simulink model "VehicleDynamicsRing"  (R2020a)
settings: Solver=FixedStepDiscrete  StartTime=0.0  StopTime=10.0  FixedStep=ModelSimTime  RelTol=1e-3  EnableMultiTasking=on
PostLoadFcn:
  | , if any(exist('dsrtsu_mdlpostloadfcn', 'file') ~= 0), dsrtsu_mdlpostloadfcn('Execute', bdroot); end,
InitFcn:
  | , if any(exist('rtifpga_mdlclblib', 'file') ~= 0), rtifpga_mdlclblib('Init', bdroot); end,
undefined symbols (not defined in the file): DRIVE_MODE, VDR
libraries: simulink x4
(part 2 of 2)

== stateflow chart VehicleDynamicsRing/VDR Mode Selection1 ==
  state VDR_MASTER
    state MODES [parallel]
      settings: executionOrder=1
      state OFF
        during:
        TVEnable = 0;
        UnstblEnable = 0;
        OpenDiffEnable = 0;
        AWDEnable = 0;
        FWDEnable = 0;
        RWDEnable = 0 ;
        MotorStatus = [0,0,0,0];
        DriveEnable = 0;
        StartUpTest = 0;
        Status = VDR.OFF;
        APPS_Status = VDR.ERROR.APPS.OKAY;
      state STARTUP
        entry:
        StartUpTestCheck();
        TVEnable = 1;
        UnstblEnable = 1;
        OpenDiffEnable = 1;
        AWDEnable = 1;
        FWDEnable = 1;
        RWDEnable = 1;
        MotorStatus = [1,1,1,1];
        Status = VDR.STARTUP;
      state SHUTDOWN
        entry:
        DriveEnable = 0;
        Status = VDR.SHUTDOWN;
      state DRIVING
        entry:
        DriveEnable = 1;
        Status = VDR.DRIVING;
      (default) -> OFF
      OFF -> STARTUP : E_StartUp
      SHUTDOWN -> OFF : E_Off
      STARTUP -> SHUTDOWN [order 2] : E_FailStartUp
      DRIVING -> SHUTDOWN : E_ShutDown
      STARTUP -> DRIVING [order 1] : E_Driving
    state CHECKING_SENSORS_ERRORS_AND_DIAGNOSTICS [parallel]
      settings: executionOrder=2
      state WAITING_TO_CHECK_SENSORS
        entry:
      state CHECKING_SENSORS
        during:
        CheckingSensorsTable();
      (default) -> WAITING_TO_CHECK_SENSORS
      WAITING_TO_CHECK_SENSORS -> CHECKING_SENSORS : E_Driving
    state MODE_SELECTION_LOGIC [parallel]
      settings: executionOrder=3
      state STANDBY
        entry:
      state CHECK_MODE_CHANGE
        %Check for valid mode
      state VALID_MODE
      state CHANGE_MAIN_MODE
        entry:
        ChangeMainMode();
      state DENY_DRIVING_MODE
        entry:
        %Cannot start driving the vehicle yet
        %First need to startup the car and run tests.
        %Send out status
      state VALID_DRIVING_MODE
      state DENY_DRIVING_MODE_CHANGE1
        %Envalid mode status
      state CHECK_DRIVING_MODE_CHANGE
      state DENY_DRIVING_MODE_CHANGE
        entry: %Deny and send out status
      state APPROVED_DRIVING_MODE_CHANGE
        entry: ChangeDrivingMode();
      state DriveModeCheck = ModeChecking [function]
        (junction 1413) -> (junction 1412)
        (junction 1412) -> (junction 1414)
        (junction 1417) -> (junction 1413) [order 3] : {ModeCheck = 0;}
            | %Else Deny
        (junction 1415) -> (junction 1414) [order 2]
        (junction 1416) -> (junction 1415) [order 1] : [sum(VDRMode == 10:12) == 1]
            | %Unstable Torque Vectoring
        (junction 1417) -> (junction 1416) [order 2] : [TVEnable == 1 && sum(VDRMode == 10:15) == 1]
            | %Torque Vecoting Check
        (default) -> (junction 1417) : %START
        (junction 1416) -> (junction 1418) [order 2] : %Else Stable Torque Vectoring
        (junction 1414) -> (junction 1426)
        (junction 1415) -> (junction 1418) [order 1] : [UnstblEnable == 1]
        (junction 1417) -> (junction 1419) [order 1] : [OpenDiffEnable == 1 && sum(VDRMode == 16:18) == 1]
            | %Open Differential Check
        (junction 1419) -> (junction 1418)
        (junction 1418) -> (junction 1420) : % Main Mode  request check passed
            | % Checking for drivetrain request
        (junction 1420) -> (junction 1421) [order 1] : [VDRMode == 10 || VDRMode == 13 || VDRMode == 16 && AWDEnable == 1]
            | %Checking for AWD
        (junction 1420) -> (junction 1422) [order 2]
        (junction 1421) -> (junction 1430) : {ModeCheck = 1;}
        (junction 1422) -> (junction 1423) [order 1] : [VDRMode == 11 || VDRMode == 14 || VDRMode == 17 && FWDEnable == 1]
            | %Checking for FWD
        (junction 1422) -> (junction 1424) [order 2]
        (junction 1423) -> (junction 1429) : {ModeCheck=1;}
        (junction 1424) -> (junction 1425) [order 1] : [VDRMode == 12 || VDRMode == 15 || VDRMode == 18 && RWDEnable == 1]
            | %Checking for FWD
        (junction 1424) -> (junction 1427) [order 2] : {ModeCheck=0;}
            | %Deny
        (junction 1425) -> (junction 1428) : {ModeCheck=1;}
        (junction 1426) -> (junction 1427) : {ModeCheck = 0}
            | %Else Deny
        (junction 1428) -> (junction 1427)
        (junction 1429) -> (junction 1428)
        (junction 1430) -> (junction 1429)
        (junction 1427) -> (junction 1431) : {DriveModeCheck = ModeCheck;}
            | %END
      state CheckStatus = ValidModeChecking [function]
        (default) -> (junction 1388) : %START
            | %Checking for a valid main mode
        (junction 1388) -> (junction 1389) [order 1] : [sum(VDRMode == 0:3) == 1]
            | %Check for main modes
        (junction 1388) -> (junction 1390) [order 2]
        (junction 1389) -> (junction 1395) : {ValidModeCheck=1;}
        (junction 1390) -> (junction 1391) [order 1] : [sum(VDRMode == 10:18) == 1]
            | %Check for driving modes
        (junction 1390) -> (junction 1392) [order 2] : {ValidModeCheck=0;}
            | %Else: Invalid Mode
        (junction 1391) -> (junction 1394) : {ValidModeCheck=1;}
        (junction 1393) -> (junction 1392)
        (junction 1394) -> (junction 1393)
        (junction 1395) -> (junction 1394)
        (junction 1392) -> (junction 1396) : {CheckStatus =ValidModeCheck; }
            | %END
      (junction 982) -> (junction 983)
      (junction 983) -> STANDBY
      (junction 981) -> (junction 982)
      (default) -> STANDBY
      CHECK_MODE_CHANGE -> VALID_MODE [order 1] : [ValidModeChecking()]
      VALID_MODE -> CHANGE_MAIN_MODE [order 2]
      CHANGE_MAIN_MODE -> (junction 981)
      STANDBY -> CHECK_MODE_CHANGE : [hasChanged(VDRMode)]
      (junction 980) -> (junction 981)
      CHECK_MODE_CHANGE -> DENY_DRIVING_MODE_CHANGE1 [order 2]
      VALID_MODE -> VALID_DRIVING_MODE [order 1] : [sum(VDRMode == 10:18) ==1]
      VALID_DRIVING_MODE -> DENY_DRIVING_MODE [order 2]
      DENY_DRIVING_MODE -> (junction 980)
      (junction 979) -> (junction 980)
      VALID_DRIVING_MODE -> CHECK_DRIVING_MODE_CHANGE [order 1] : [StartUpTest == 1]
      CHECK_DRIVING_MODE_CHANGE -> DENY_DRIVING_MODE_CHANGE [order 2]
      DENY_DRIVING_MODE_CHANGE -> (junction 979)
      (junction 984) -> (junction 979)
      CHECK_DRIVING_MODE_CHANGE -> APPROVED_DRIVING_MODE_CHANGE [order 1] : [ModeChecking()]
      APPROVED_DRIVING_MODE_CHANGE -> (junction 984)
    state MOTOR_STATUSES [parallel]
      entry:
      encoder_torque_counter_FL = 0;
      encoder_torque_counter_FR = 0;
      encoder_torque_counter_RL = 0;
      encoder_torque_counter_RR = 0;
      acceleration_torque_counter_FL = 0;
      acceleration_torque_counter_FR = 0;
      acceleration_torque_counter_RL = 0;
      acceleration_torque_counter_RR = 0;
      settings: executionOrder=4
      state MOTOR_STATUS_FL [parallel] [commented out]
        state MOTOR_CHECKING_FL [commented out]
          state MOTOR_ENCODER_CHECK_FL [parallel] [commented out]
            state CHECKING_ENC_FL [commented out]
              during:
              encoder_torque_counter_FL = duration_encoder_torque_check(SystemTrqCmd ,Encoder_FL,encoder_torque_counter_FL);
            state ENC_ERR_FL [commented out]
              en:
              send(E_MtrErrFL,MOTOR_STATUS_FL)
            (default) -> CHECKING_ENC_FL [commented out]
            CHECKING_ENC_FL -> ENC_ERR_FL [commented out] : [encoder_torque_counter_FL >= VDR.EncoderTorqueCounter]
          state MOTOR_ACCEL_CHECK_FL [parallel] [commented out]
            state ERR_ACCEL_FL [commented out]
              en:
              send(E_MtrErrFL,MOTOR_STATUS_FL)
            state CHECKING_ACCEL_FL [commented out]
              during:
              acceleration_torque_counter_FL = duration_acceleration_torque_check(SystemTrqCmd ,Accel_X,acceleration_torque_counter_FL);
            (default) -> CHECKING_ACCEL_FL [commented out]
            CHECKING_ACCEL_FL -> ERR_ACCEL_FL [commented out] : [acceleration_torque_counter_FL >= VDR.AccelTorqueCounter]
          state MOTOR_TRQ_LIMIT_CHECK_FL [parallel] [commented out]
            state CHECKING_TRQ_LIMIT_FL [commented out]
            state ERR_TRQ_LIMIT_FL [commented out]
              en:
              send(E_MtrErrFL,MOTOR_STATUS_FL)
            (default) -> CHECKING_TRQ_LIMIT_FL [commented out]
            CHECKING_TRQ_LIMIT_FL -> ERR_TRQ_LIMIT_FL [commented out] : [TorqueLimit_FL > 21 || TorqueLimit_FL < 0]
          state MOTOR_ENCODER_VALUE_CHECK_FL [parallel] [commented out]
            state CHECKING_ENCODER_VALUE_FL [commented out]
            state ERR_ENCODER_VALUEL_FL [commented out]
              en:
              send(E_MtrErrFL,MOTOR_STATUS_FL)
            (default) -> CHECKING_ENCODER_VALUE_FL [commented out]
            CHECKING_ENCODER_VALUE_FL -> ERR_ENCODER_VALUEL_FL [commented out] : [Encoder_FL > 7000]
        state FWD_OFF_FL [commented out]
          entry:
          %nothing
        state MTR_ERR_FL [commented out]
          entry:
          %send status
          FWDEnable = 0;
        (default) -> MOTOR_CHECKING_FL [commented out]
        MOTOR_CHECKING_FL -> FWD_OFF_FL [commented out] : [FWDEnable == 0]
        MOTOR_CHECKING_FL -> MTR_ERR_FL [commented out] : E_MtrErrFL
      state MOTOR_STATUS_FR [parallel] [commented out]
        state MOTOR_CHECKING_FR [commented out]
          state MOTOR_ENCODER_CHECK_FR [parallel] [commented out]
            state CHECKING_ENC_FR [commented out]
              during:
              encoder_torque_counter_FR = duration_encoder_torque_check(SystemTrqCmd ,Encoder_FR,encoder_torque_counter_FR);
            state ENC_ERR_FR [commented out]
              en:
              send(E_MtrErrFR,MOTOR_STATUS_FR)
            (default) -> CHECKING_ENC_FR [commented out]
            CHECKING_ENC_FR -> ENC_ERR_FR [commented out] : [encoder_torque_counter_FR >= VDR.EncoderTorqueCounter]
          state MOTOR_ACCEL_CHECK_FR [parallel] [commented out]
            state ERR_ACCEL_FR [commented out]
              en:
              send(E_MtrErrFR,MOTOR_STATUS_FR)
            state CHECKING_ACCEL_FR [commented out]
              during:
              acceleration_torque_counter_FR = duration_acceleration_torque_check(SystemTrqCmd ,Accel_X,acceleration_torque_counter_FR);
            (default) -> CHECKING_ACCEL_FR [commented out]
            CHECKING_ACCEL_FR -> ERR_ACCEL_FR [commented out] : [acceleration_torque_counter_FR >= VDR.AccelTorqueCounter]
          state MOTOR_TRQ_LIMIT_CHECK_FR [parallel] [commented out]
            state CHECKING_TRQ_LIMIT_FR [commented out]
            state ERR_TRQ_LIMIT_FR [commented out]
              en:
              send(E_MtrErrFR,MOTOR_STATUS_FR)
            (default) -> CHECKING_TRQ_LIMIT_FR [commented out]
            CHECKING_TRQ_LIMIT_FR -> ERR_TRQ_LIMIT_FR [commented out] : [TorqueLimit_FR > 21 || TorqueLimit_FR < 0]
          state MOTOR_ENCODER_VALUE_CHECK_FR [parallel] [commented out]
            state CHECKING_ENCODER_VALUE_FR [commented out]
            state ERR_ENCODER_VALUEL_FR [commented out]
              en:
              send(E_MtrErrFR,MOTOR_STATUS_FR)
            (default) -> CHECKING_ENCODER_VALUE_FR [commented out]
            CHECKING_ENCODER_VALUE_FR -> ERR_ENCODER_VALUEL_FR [commented out] : [Encoder_FR > 7000]
        state FWD_OFF_FR [commented out]
          entry:
          %nothing
        state MTR_ERR_FR [commented out]
          entry:
          %send status
          FWDEnable = 0;
        (default) -> MOTOR_CHECKING_FR [commented out]
        MOTOR_CHECKING_FR -> FWD_OFF_FR [commented out] : [FWDEnable == 0]
        MOTOR_CHECKING_FR -> MTR_ERR_FR [commented out] : E_MtrErrFR
      state MOTOR_STATUS_RL [parallel] [commented out]
        state MOTOR_CHECKING_RL [commented out]
          state MOTOR_ENCODER_CHECK_RL [parallel] [commented out]
            state CHECKING_ENC_RL [commented out]
              during:
              encoder_torque_counter_RL = duration_encoder_torque_check(SystemTrqCmd ,Encoder_RL,encoder_torque_counter_RL);
            state ENC_ERR_RL [commented out]
              en:
              send(E_MtrErrRL,MOTOR_STATUS_RL)
            (default) -> CHECKING_ENC_RL [commented out]
            CHECKING_ENC_RL -> ENC_ERR_RL [commented out] : [encoder_torque_counter_RL >= VDR.EncoderTorqueCounter]
          state MOTOR_ACCEL_CHECK_RL [parallel] [commented out]
            state ERR_ACCEL_RL [commented out]
              en:
              send(E_MtrErrRL,MOTOR_STATUS_RL)
            state CHECKING_ACCEL_RL [commented out]
              during:
              acceleration_torque_counter_RL = duration_acceleration_torque_check(SystemTrqCmd ,Accel_X,acceleration_torque_counter_RL);
            (default) -> CHECKING_ACCEL_RL [commented out]
            CHECKING_ACCEL_RL -> ERR_ACCEL_RL [commented out] : [acceleration_torque_counter_RL >= VDR.AccelTorqueCounter]
          state MOTOR_TRQ_LIMIT_CHECK_RL [parallel] [commented out]
            state CHECKING_TRQ_LIMIT_RL [commented out]
            state ERR_TRQ_LIMIT_RL [commented out]
              en:
              send(E_MtrErrRL,MOTOR_STATUS_RL)
            (default) -> CHECKING_TRQ_LIMIT_RL [commented out]
            CHECKING_TRQ_LIMIT_RL -> ERR_TRQ_LIMIT_RL [commented out] : [TorqueLimit_RL > 21 || TorqueLimit_RL < 0]
          state MOTOR_ENCODER_VALUE_CHECK_RL [parallel] [commented out]
            state CHECKING_ENCODER_VALUE_RL [commented out]
            state ERR_ENCODER_VALUEL_RL [commented out]
              en:
              send(E_MtrErrRL,MOTOR_STATUS_RL)
            (default) -> CHECKING_ENCODER_VALUE_RL [commented out]
            CHECKING_ENCODER_VALUE_RL -> ERR_ENCODER_VALUEL_RL [commented out] : [Encoder_RL > 7000]
        state FWD_OFF_RL [commented out]
          entry:
          %nothing
        state MTR_ERR_RL [commented out]
          entry:
          %send status
          FWDEnable = 0;
        (default) -> MOTOR_CHECKING_RL [commented out]
        MOTOR_CHECKING_RL -> FWD_OFF_RL [commented out] : [FWDEnable == 0]
        MOTOR_CHECKING_RL -> MTR_ERR_RL [commented out] : E_MtrErrRL
      state MOTOR_STATUS_RR [parallel] [commented out]
        state MOTOR_CHECKING_RR [commented out]
          state MOTOR_ENCODER_CHECK_RR [parallel] [commented out]
            state CHECKING_ENC_RR [commented out]
              during:
              encoder_torque_counter_RR = duration_encoder_torque_check(SystemTrqCmd ,Encoder_RR,encoder_torque_counter_RR);
            state ENC_ERR_RR [commented out]
              en:
              send(E_MtrErrRR,MOTOR_STATUS_RR)
            (default) -> CHECKING_ENC_RR [commented out]
            CHECKING_ENC_RR -> ENC_ERR_RR [commented out] : [encoder_torque_counter_RR >= VDR.EncoderTorqueCounter]
          state MOTOR_ACCEL_CHECK_RR [parallel] [commented out]
            state ERR_ACCEL_RR [commented out]
              en:
              send(E_MtrErrRR,MOTOR_STATUS_RR)
            state CHECKING_ACCEL_RR [commented out]
              during:
              acceleration_torque_counter_RR = duration_acceleration_torque_check(SystemTrqCmd ,Accel_X,acceleration_torque_counter_RR);
            (default) -> CHECKING_ACCEL_RR [commented out]
            CHECKING_ACCEL_RR -> ERR_ACCEL_RR [commented out] : [acceleration_torque_counter_RR >= VDR.AccelTorqueCounter]
          state MOTOR_TRQ_LIMIT_CHECK_RR [parallel] [commented out]
            state CHECKING_TRQ_LIMIT_RR [commented out]
            state ERR_TRQ_LIMIT_RR [commented out]
              en:
              send(E_MtrErrRR,MOTOR_STATUS_RR)
            (default) -> CHECKING_TRQ_LIMIT_RR [commented out]
            CHECKING_TRQ_LIMIT_RR -> ERR_TRQ_LIMIT_RR [commented out] : [TorqueLimit_RR > 21 || TorqueLimit_RR < 0]
          state MOTOR_ENCODER_VALUE_CHECK_RR [parallel] [commented out]
            state CHECKING_ENCODER_VALUE_RR [commented out]
            state ERR_ENCODER_VALUEL_RR [commented out]
              en:
              send(E_MtrErrRR,MOTOR_STATUS_RR)
            (default) -> CHECKING_ENCODER_VALUE_RR [commented out]
            CHECKING_ENCODER_VALUE_RR -> ERR_ENCODER_VALUEL_RR [commented out] : [Encoder_RR > 7000]
        state FWD_OFF_RR [commented out]
          entry:
          %nothing
        state MTR_ERR_RR [commented out]
          entry:
          %send status
          FWDEnable = 0;
        (default) -> MOTOR_CHECKING_RR [commented out]
        MOTOR_CHECKING_RR -> FWD_OFF_RR [commented out] : [FWDEnable == 0]
        MOTOR_CHECKING_RR -> MTR_ERR_RR [commented out] : E_MtrErrRR
      state updated_counter = duration_encoder_torque_check(trq,encoder,counter) [function]
      state updated_counter = duration_acceleration_torque_check(trq,accel,counter) [function]
  (default) -> VDR_MASTER
  data: DriveModeCheck function_output; CheckStatus function_output; trq function_input double size=1; encoder function_input double size=1; counter function_input double size=1; updated_counter function_output; trq function_input double size=1; accel function_input double size=1; counter function_input double size=1; updated_counter function_output; VDRMode input; VDR parameter; TVEnable local; UnstblEnable local; OpenDiffEnable local; AWDEnable local; FWDEnable local; RWDEnable local; MotorStatus local; APPS1 input; APPS2 input; Accel_X input; Accel_Y input; Speed_X input; Speed input; SteerAngle input; APPS input; Encoder_FL input; Encoder_FR input; Encoder_RL input; Encoder_RR input; SystemTrqCmd input; TorqueLimit_FL input; TorqueLimit_FR input; TorqueLimit_RL input; TorqueLimit_RR input; ValidModeCheck local; encoder_torque_counter_FL local double; acceleration_torque_counter_FL local double; acceleration_torque_counter_RL local double; acceleration_torque_counter_RR local double; encoder_torque_counter_RR local double; encoder_torque_counter_FR local double; encoder_torque_counter_RL local double; acceleration_torque_counter_FR local double; DrivingMode output; TVControl output; Drivetrain output; DriveEnable output; Status output; APPS_Status output; StartUpTest local
  events: E_StartUp local FUNCTION_CALL_EVENT; E_ShutDown local FUNCTION_CALL_EVENT; E_Off local FUNCTION_CALL_EVENT; E_FailStartUp local FUNCTION_CALL_EVENT; E_Driving local FUNCTION_CALL_EVENT; E_MtrErrRR local FUNCTION_CALL_EVENT; E_MtrErrFL local FUNCTION_CALL_EVENT; E_MtrErrFR local FUNCTION_CALL_EVENT; E_MtrErrRL local FUNCTION_CALL_EVENT; E_CommunicationCheck local RISING_EDGE_EVENT
  function StartUpTestCheck:
    | function StartUpTestCheck
    | 
    | aVarTruthTableCondition_1 = false;
    | aVarTruthTableCondition_2 = false;
    | aVarTruthTableCondition_3 = false;
    | aVarTruthTableCondition_4 = false;
    | aVarTruthTableCondition_5 = false;
    | aVarTruthTableCondition_6 = false;
    | 
    | 
    | % Look at APPS
    | 
    | aVarTruthTableCondition_1 = logical(APPS >= 0 && APPS <= 100);
    | 
    | % Car is not moving check: accel-x
    | 
    | aVarTruthTableCondition_2 = logical(abs(Accel_X) < VDR.MinAccelX);
    | 
    | % Car is not moving check: accel-y
    | 
    | aVarTruthTableCondition_3 = logical(abs(Accel_Y) < VDR.MinAccelY);
    | 
    | % Velocity-x sensor is zero
    | 
    | aVarTruthTableCondition_4 = logical(abs(Speed_X) < VDR.MinVelocityX);
    | 
    | % Velocity sensor is zero
    | 
    | aVarTruthTableCondition_5 = logical(abs(Speed) < VDR.MinVelocity);
    | 
    | % Check Steering Wheel calibr.
    | 
    | aVarTruthTableCondition_6 = logical(abs(SteerAngle) < VDR.MaxSteerAngle);
    | 
    | if (aVarTruthTableCondition_1 && aVarTruthTableCondition_2 && aVarTruthTableCondition_3 && aVarTruthTableCondition_4 && aVarTruthTableCondition_5 && aVarTruthTableCondition_6)
    |     aFcnTruthTableAction_1();
    | else % Default
    |     aFcnTruthTableAction_2();
    | end
    | 
    | function aFcnTruthTableAction_1()
    | 
    | % The car is stationary and can now be started up.
    | 
    | StartUpTest = 1;
    | 
    | function aFcnTruthTableAction_2()
    | 
    | % The car sensors readons are incorrect or the car is moving. So the car should not be started up.
    | 
    | send(E_FailStartUp,MODES);
  function CheckingSensorsTable:
    | function CheckingSensorsTable
    | 
    | aVarTruthTableCondition_1 = false;
    | aVarTruthTableCondition_2 = false;
    | aVarTruthTableCondition_3 = false;
    | aVarTruthTableCondition_4 = false;
    | aVarTruthTableCondition_5 = false;
    | 
    | 
    | % Steering sensor sanity check
    | 
    | aVarTruthTableCondition_1 = logical(abs(SteerAngle) > VDR.MaxSteerAngle);
    | 
    | % System Command Torque Check
    | 
    | aVarTruthTableCondition_2 = logical(abs(SystemTrqCmd) > 90);
    | 
    | % APPS competition requirements
    | 
    | aVarTruthTableCondition_3 = logical(abs(APPS1 - APPS2)/APPS1 >= 0.1);
    | 
    | % Accelerator-x sanity check
    | 
    | aVarTruthTableCondition_4 = logical(abs(Accel_X) > VDR.MaxAccelX);
    | 
    | % Accelerator-y sanity check
    | 
    | aVarTruthTableCondition_5 = logical(abs(Accel_Y) > VDR.MaxAccelY);
    | 
    | if (aVarTruthTableCondition_1)
    |     aFcnTruthTableAction_1();
    |     aFcnTruthTableAction_3();
    | elseif (aVarTruthTableCondition_2)
    |     aFcnTruthTableAction_1();
    | elseif (aVarTruthTableCondition_3)
    |     aFcnTruthTableAction_1();
    |     aFcnTruthTableAction_2();
    | elseif (aVarTruthTableCondition_4)
    |     aFcnTruthTableAction_3();
    | elseif (aVarTruthTableCondition_5)
    |     aFcnTruthTableAction_3();
    | else % Default
    |     aFcnTruthTableAction_1();
    | end
    | 
    | function aFcnTruthTableAction_1()
    | 
    | % Impossible and/or out of range values. Must shutdown the vehicle.
    | 
    | send(E_ShutDown,MODES);
    | 
    | function aFcnTruthTableAction_2()
    | 
    | % APPS Failure
    | 
    | APPS_Status = VDR.ERROR.APPS.FAILURE;
    | 
    | function aFcnTruthTableAction_3()
    | 
    | % Disable the unstable Torque Vectoring controller
    | 
    | UnstblEnable = 0;
  function ChangeMainMode:
    | function ChangeMainMode
    | switch(VDRMode)
    |     case VDR.Mode.OFF
    |         send(E_Off,MODES);
    |     case VDR.Mode.STARTUP
    |         send(E_StartUp,MODES);
    |     case VDR.Mode.DRIVING
    |         send(E_Driving,MODES);
    |     case VDR.Mode.SHUTDOWN
    |         send(E_ShutDown,MODES);
    |     otherwise
    |         send(E_ShutDown,MODES);
    | end
  function ChangeMainMode12:
    | function ChangeMainMode12
    | 
    | aVarTruthTableCondition_1 = false;
    | aVarTruthTableCondition_2 = false;
    | aVarTruthTableCondition_3 = false;
    | aVarTruthTableCondition_4 = false;
    | 
    | 
    | % Startup requested
    | 
    | aVarTruthTableCondition_1 = logical(VDRMode == 0);
    | 
    | % Shutdown requested
    | 
    | aVarTruthTableCondition_2 = logical(VDRMode == 1);
    | 
    | % Driving requested
    | 
    | aVarTruthTableCondition_3 = logical(VDRMode == 2);
    | 
    | % OFF requested
    | 
    | aVarTruthTableCondition_4 = logical(VDRMode == 3);
    | 
    | if (aVarTruthTableCondition_1)
    |     aFcnTruthTableAction_1();
    | elseif (aVarTruthTableCondition_2)
    |     aFcnTruthTableAction_2();
    | elseif (aVarTruthTableCondition_3)
    |     aFcnTruthTableAction_3();
    | elseif (aVarTruthTableCondition_4)
    |     aFcnTruthTableAction_4();
    | else % Default
    |     aFcnTruthTableAction_4();
    | end
    | 
    | function aFcnTruthTableAction_1()
    | 
    | % Switch to Startup
    | 
    | send(E_StartUp,MODES);
    | 
    | function aFcnTruthTableAction_2()
    | 
    | % Switch to Shutdown
    | 
    | send(E_Off,MODES);
    | 
    | function aFcnTruthTableAction_3()
    | 
    | % Switch to OFF
    | 
    | send(E_Driving,MODES);
    | 
    | function aFcnTruthTableAction_4()
    | 
    | % Error in mode selection.
    | 
    | send(E_ShutDown,MODES);
  function ChangeDrivingMode:
    | function ChangeDrivingMode
    | 
    | aVarTruthTableCondition_1 = false;
    | aVarTruthTableCondition_2 = false;
    | aVarTruthTableCondition_3 = false;
    | aVarTruthTableCondition_4 = false;
    | aVarTruthTableCondition_5 = false;
    | aVarTruthTableCondition_6 = false;
    | aVarTruthTableCondition_7 = false;
    | aVarTruthTableCondition_8 = false;
    | aVarTruthTableCondition_9 = false;
    | 
    | 
    | % Torque Vecotring Unstable AWD requested
    | 
    | aVarTruthTableCondition_1 = logical(VDRMode == 10);
    | 
    | % Torque Vecotring Unstable FWD requested
    | 
    | aVarTruthTableCondition_2 = logical(VDRMode == 11);
    | 
    | % Torque Vecotring Unstable RWD requested
    | 
    | aVarTruthTableCondition_3 = logical(VDRMode == 12);
    | 
    | % Torque Vecotring Stable AWD requested
    | 
    | aVarTruthTableCondition_4 = logical(VDRMode == 13);
    | 
    | % Torque Vecotring Stable FWD requested
    | 
    | aVarTruthTableCondition_5 = logical(VDRMode == 14);
    | 
    | % Torque Vecotring Stable RWD requested
    | 
    | aVarTruthTableCondition_6 = logical(VDRMode == 15);
    | 
    | % Open Differential AWD requested
    | 
    | aVarTruthTableCondition_7 = logical(VDRMode == 16);
    | 
    | % Open Differential FWD requested
    | 
    | aVarTruthTableCondition_8 = logical(VDRMode == 17);
    | 
    | % Open Differential RWD
    | % requested
    | 
    | aVarTruthTableCondition_9 = logical(VDRMode == 18);
    | 
    | if (aVarTruthTableCondition_1)
    |     aFcnTruthTableAction_1();
    | elseif (aVarTruthTableCondition_2)
    |     aFcnTruthTableAction_2();
    | elseif (aVarTruthTableCondition_3)
    |     aFcnTruthTableAction_3();
    | elseif (aVarTruthTableCondition_4)
    |     aFcnTruthTableAction_4();
    | elseif (aVarTruthTableCondition_5)
    |     aFcnTruthTableAction_5();
    | elseif (aVarTruthTableCondition_6)
    |     aFcnTruthTableAction_6();
    | elseif (aVarTruthTableCondition_7)
    |     aFcnTruthTableAction_7();
    | elseif (aVarTruthTableCondition_8)
    |     aFcnTruthTableAction_8();
    | elseif (aVarTruthTableCondition_9)
    |     aFcnTruthTableAction_9();
    | else % Default
    |     aFcnTruthTableAction_10();
    | end
    | 
    | function aFcnTruthTableAction_1()
    | 
    | % Switch to Torque Vecotring Unstable AWD
    | 
    | DrivingMode = 1;
    | TVControl = 1;
    | Drivetrain = 2;
    | 
    | function aFcnTruthTableAction_2()
    | 
    | % Switch to Torque Vecotring Unstable FWD
    | 
    | DrivingMode = 1;
    | TVControl = 1;
    | Drivetrain = 1;
    | 
    | function aFcnTruthTableAction_3()
    | 
    | % Switch to Torque Vecotring Unstable RWD
    | 
    | DrivingMode = 1;
    | TVControl = 1;
    | Drivetrain = 0;
    | 
    | function aFcnTruthTableAction_4()
    | 
    | % Switch to Torque Vecotring Stable AWD
    | 
    | DrivingMode = 1;
    | TVControl = 0;
    | Drivetrain = 2;
    | 
    | function aFcnTruthTableAction_5()
    | 
    | % Switch to Torque Vecotring Stable FWD
    | 
    | DrivingMode = 1;
    | TVControl = 0;
    | Drivetrain = 1;
    | 
    | function aFcnTruthTableAction_6()
    | 
    | % Switch to Torque Vecotring Stable RWD
    | 
    | DrivingMode = 1;
    | TVControl = 0;
    | Drivetrain = 0;
    | 
    | function aFcnTruthTableAction_7()
    | 
    | % Switch to Open Differential AWD
    | 
    | DrivingMode = 1;
    | Drivetrain = 2;
    | 
    | function aFcnTruthTableAction_8()
    | 
    | % Switch to Open Differential FWD
    | 
    | DrivingMode = 1;
    | Drivetrain = 1;
    | 
    | function aFcnTruthTableAction_9()
    | 
    | % Switch to Open Differential RWD
    | 
    | DrivingMode = 1;
    | Drivetrain = 0;
    | 
    | function aFcnTruthTableAction_10()
    | 
    | % Error in mode selection.
    | 
    | send(E_ShutDown,MODES);

== matlab function VehicleDynamicsRing/torque_distribution_mapping ==
  data: systemTorque input; torqueFactors input size=4; torqueRequests output Bus: TorqueRequests; torqueLimits input Bus: TorqueLimits; driveEnabled input
function torqueRequests = torque_vectoring(systemTorque,torqueFactors,torqueLimits, driveEnabled)
% This function calculates the optimal torque distribution based on the
% relative torque scaling factors (determined by vehicle acceleration and
% understeering/oversteering) and the torque limits for each motor.
% torque_scales: fl, fr, rl, rr
% torque_limits: fl, fr, rl, rr

% Optimal torque distribution is determined by maintaining the relative
% torque scaling factors and using a nominal torque such that system torque
% is maximized and the torque limits for all motors are not exceeded

% Ex: Torque_fl = torque_scales[1]*torque_nominal

torqueRequests.TorqueFrontLeft = 0;
torqueRequests.TorqueFrontRight = 0;
torqueRequests.TorqueRearLeft = 0;
torqueRequests.TorqueRearRight = 0;
nominalTorque = systemTorque/4;
tempNominalTorque = [nominalTorque,nominalTorque,nominalTorque,nominalTorque];

if(driveEnabled)
    if(torqueFactors(1) ~= 0)
        tempNominalTorque(1) = torqueLimits.TorqueLimitFrontLeft/torqueFactors(1);
    end
    if(torqueFactors(2) ~= 0)
        tempNominalTorque(2) = torqueLimits.TorqueLimitFrontRight/torqueFactors(2);
    end
    if(torqueFactors(3) ~= 0)
        tempNominalTorque(3) = torqueLimits.TorqueLimitRearLeft/torqueFactors(3);
    end
    if(torqueFactors(4) ~= 0)
        tempNominalTorque(4) = torqueLimits.TorqueLimitRearRight/torqueFactors(4);
    end
    
    nominalTorque = min(tempNominalTorque);
  
    torqueRequests.TorqueFrontLeft = nominalTorque * torqueFactors(1);
    torqueRequests.TorqueFrontRight = nominalTorque * torqueFactors(2);
    torqueRequests.TorqueRearLeft = nominalTorque * torqueFactors(3);
    torqueRequests.TorqueRearRight = nominalTorque * torqueFactors(4);
    
end
end

% torque_requests = [0,0,0,0];
% torque_nominal = 0;
% total_system_torque = 0;
% temp_system_torque = 0;
% limit_fail = false;

% for i = 1:size(torque_scales)
%     limit_fail = false;
%     temp_system_torque = 0;
%     temp_nominal = torque_limits[i]/torque_scales[i];
%     for j = 1:size(torque_scales)
%         if(temp_nominal*torque_scales[j] > torque_limits[j])
%             limit_fail = true;
%             break;
%         end
%         temp_system_torque = temp_system_torque + temp_nominal*torque_scales[j];
%     end
%     if(limit_fail)
%         continue;
%     end
%     if(temp_system_torque > total_system_torque)
%         total_system_torque = temp_system_torque;
%         torque_nominal = temp_nominal;
%     end
% end
% 
% for i = 1:size(torque_scales)
%     torque_requests[i] = torque_nominal*torque_scales[i];
% end
% 
% end %done

== stateflow chart VehicleDynamicsRing/VDR Mode Selection ==
  state OFF
    during:
    TorqueVectoringUnstableEnabled = false;
    DriveEnabled = false;
    TorqueVectoringStableEnabled = false;
    VdrStatus = RING_STATUS.OFF;
  state SHUTDOWN
    entry:
    VdrStatus = RING_STATUS.SHUTDOWN_IN_PROGRESS_HV;
    %TODO: Add checks for shutdown
    VdrStatus = RING_STATUS.SHUTDOWN_COMPLETE_HV;
  state OPERATIONAL
    state STARTUP
      entry:
      VdrStatus = RING_STATUS.STARTUP_IN_PROGRESS_HV;
    state RUNNING
      entry:
      DriveEnabled = true;
      VdrStatus = RING_STATUS.RUNNING;
      exit:
      DriveEnabled = false;
      state DRIVING_MODE
      state TORQUE_VECTORING
        state CHECK_TORQUE_VECTORING_MODE
        state TORQUE_VECTORING_UNSTABLE
          entry:
          TorqueVectoringUnstableEnabled = true;
          exit:
          TorqueVectoringUnstableEnabled = false;
        state TORQUE_VECTORING_STABLE
          entry:
          TorqueVectoringStableEnabled = true;
          exit:
          TorqueVectoringStableEnabled = false;
        (default) -> CHECK_TORQUE_VECTORING_MODE
        CHECK_TORQUE_VECTORING_MODE -> TORQUE_VECTORING_UNSTABLE [order 1] : [DrivingMode == DRIVE_MODE.TORQUE_VECTORING_STABLE]
        CHECK_TORQUE_VECTORING_MODE -> TORQUE_VECTORING_STABLE [order 2] : [DrivingMode == DRIVE_MODE.TORQUE_VECTORING_STABLE]
        TORQUE_VECTORING_UNSTABLE -> TORQUE_VECTORING_STABLE : [DrivingMode == DRIVE_MODE.TORQUE_VECTORING_STABLE]
      state TORQUE_VECTORING_STABLE1
        entry:
        OpenDifferentialEnabled = true;
        exit:
        OpenDifferentialEnabled = false;
      (default) -> DRIVING_MODE
      DRIVING_MODE -> TORQUE_VECTORING [order 1] : [DrivingMode == DRIVE_MODE.TORQUE_VECTORING_STABLE ||...
          | DrivingMode == DRIVE_MODE.TORQUE_VECTORING_STABLE]
      DRIVING_MODE -> TORQUE_VECTORING_STABLE1 [order 2] : [DrivingMode == DRIVE_MODE.OPEN_DIFFERENTIAL]
      TORQUE_VECTORING -> TORQUE_VECTORING_STABLE1 : [DrivingMode == DRIVE_MODE.OPEN_DIFFERENTIAL]
    state STARTUP_PASS
      entry:
      VdrStatus = RING_STATUS.STARTUP_COMPLETE_HV;
    (default) -> STARTUP
    STARTUP -> STARTUP_PASS
    STARTUP_PASS -> RUNNING : [VdrModeRequest == VDR.Mode.DRIVING &&...
        | VdrStatus == RING_STATUS.STARTUP_COMPLETE_HV]
  (default) -> OFF
  OPERATIONAL -> SHUTDOWN : [VdrModeRequest == MSR_REQUEST.SHUTDOWN_HV]
  OFF -> OPERATIONAL : [VdrModeRequest == MSR_REQUEST.STARTUP_HV]
  data: VdrModeRequest input Enum: MSR_REQUEST; VDR parameter; DriveEnabled output boolean; OpenDifferentialEnabled output boolean; TorqueVectoringUnstableEnabled output boolean; TorqueVectoringStableEnabled output boolean; VdrStatus output Enum: RING_STATUS; DrivingMode input Enum: DRIVE_MODE
  function StartUpTestCheck:
    | function StartUpTestCheck
    | 
    | aVarTruthTableCondition_1 = false;
    | aVarTruthTableCondition_2 = false;
    | aVarTruthTableCondition_3 = false;
    | aVarTruthTableCondition_4 = false;
    | 
    | 
    | % Look at APPS
    | 
    | aVarTruthTableCondition_1 = logical(APPS >= 0 && APPS <= 100);
    | 
    | % Car is not moving check: accel-x
    | 
    | aVarTruthTableCondition_2 = logical(abs(Accel_X) < VDR.MinAccelX);
    | 
    | % Car is not moving check: accel-y
    | 
    | aVarTruthTableCondition_3 = logical(abs(Accel_Y) < VDR.MinAccelY);
    | 
    | % Velocity sensor is zero
    | 
    | aVarTruthTableCondition_4 = logical(abs(Speed) < VDR.MinVelocity);
    | 
    | if (aVarTruthTableCondition_1 && aVarTruthTableCondition_2 && aVarTruthTableCondition_3 && aVarTruthTableCondition_4)
    |     aFcnTruthTableAction_1();
    | else % Default
    |     aFcnTruthTableAction_2();
    | end
    | 
    | function aFcnTruthTableAction_1()
    | 
    | % The car is stationary and can now be started up.
    | 
    | StartUpTest = VDR.PASS;
    | 
    | function aFcnTruthTableAction_2()
    | 
    | % The car sensors readins are incorrect or the car is moving. So the car should not be started up.
    | 
    | StartUpTest = VDR.FAIL;
  function CheckingSensorsTable:
    | function CheckingSensorsTable
    | 
    | aVarTruthTableCondition_1 = false;
    | aVarTruthTableCondition_2 = false;
    | aVarTruthTableCondition_3 = false;
    | aVarTruthTableCondition_4 = false;
    | 
    | 
    | % System Command Torque Check
    | 
    | aVarTruthTableCondition_1 = logical(abs(SystemTrqCmd) > 90);
    | 
    | % APPS competition requirements
    | 
    | aVarTruthTableCondition_2 = logical(abs(APPS1 - APPS2)/APPS1 >= 0.1);
    | 
    | % Accelerator-x sanity check
    | 
    | aVarTruthTableCondition_3 = logical(abs(Accel_X) > VDR.MaxAccelX);
    | 
    | % Accelerator-y sanity check
    | 
    | aVarTruthTableCondition_4 = logical(abs(Accel_Y) > VDR.MaxAccelY);
    | 
    | if (aVarTruthTableCondition_1)
    |     aFcnTruthTableAction_1();
    | elseif (aVarTruthTableCondition_2)
    |     aFcnTruthTableAction_1();
    |     aFcnTruthTableAction_2();
    | elseif (aVarTruthTableCondition_3)
    |     aFcnTruthTableAction_1();
    | elseif (aVarTruthTableCondition_4)
    |     aFcnTruthTableAction_1();
    | else % Default
    |     aFcnTruthTableAction_3();
    | end
    | 
    | function aFcnTruthTableAction_1()
    | 
    | % Impossible and/or out of range values. Must shutdown the vehicle.
    | 
    | SensorFailure = 1;
    | 
    | function aFcnTruthTableAction_2()
    | 
    | % APPS Failure
    | 
    | APPS_Status = VDR.ERROR.APPS.FAILURE;
    | 
    | function aFcnTruthTableAction_3()
    | 
    | % DO NOTHING
  function StartUpTestFnc:
    | function StartUpTestFnc
    | temp = true;
    | if(APPS >= 0 && APPS <= 100)
    |     temp = false;
    | end
    | end
